simulink model "Simulation"  (R2021b)
settings: Solver=FixedStepAuto  StartTime=0.0  StopTime=30  FixedStep=Ts  RelTol=1e-3
InitFcn:
  | Tf = 200;
  | Ts = 0.01;
  | T = 0:Ts:Tf;
  | rolla = T';
  | omegaa=T';
  | omegax =T';
  | %%
  | 
  | load('A');
  | A = A(2001:2000+length(T),:);
  | rolla(:,2) = A(:,2)-0.0661;
  | omegaa(:,2) = A(:,1);
  | omegax(:,2) = A(:,3);
  | %%
  | l1 =10;
  | initial_vector_error = ones(1,l1)*0.001;
  | initial_vector_error(1) = 0.001;
undefined symbols (not defined in the file or in its folder): X, Y, Z
libraries: nesl_utility x23, sm_lib x15, simulink x3
(part 1 of 2)
settings Model: Creator=mirha  LastModifiedBy=Ali
settings SolverCC: AlgebraicLoopSolver=TrustRegion
settings DataIOCC: ReturnWorkspaceOutputs=off
settings DebuggingCC: SFMachineParentedDataDiag=warning  ArithmeticOperatorsInVariantConditions=warning
settings SFSimCC: SimUseLocalCustomCode=off  CustomCodeUndefinedFunction=UseInterfaceOnly
settings RTWCC: RTWUseLocalCustomCode=off

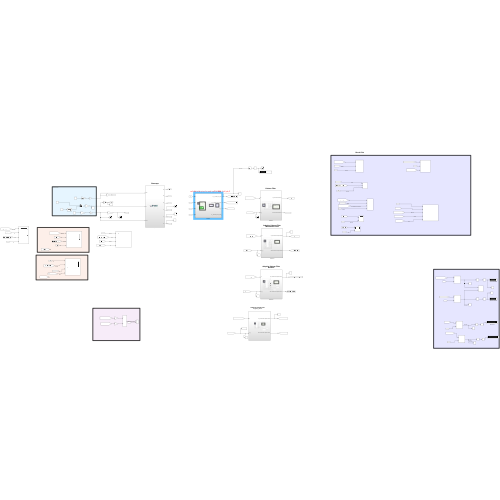
[thumbnail: Simulink's stored preview of the top-level diagram]
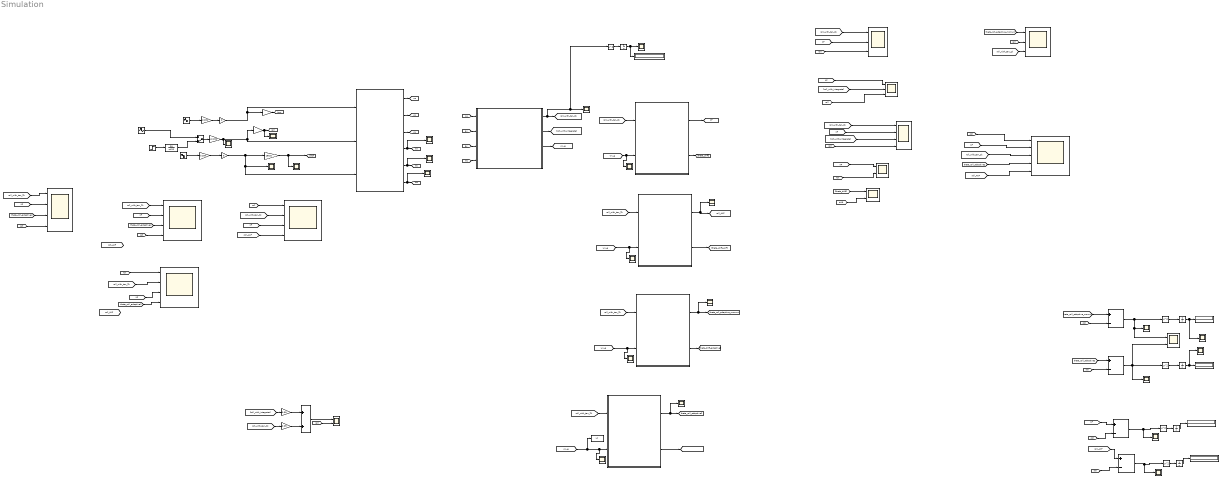
== system Simulation ==
  note: RMS error
  note: Result plot
  note: Kalman Filter
  note: اثر نویز که از IMA اندازگیری کردیم رو توی این بلوک اضافه شده
  note: plot
  note: Desired theta
  note: Result Plot
  note: Simscape
  note: Adaptive Kalman Filter
      | Momuni
  note: Adaptive Kalman Filter
      | Mohammad 1999
  note: Adaptive Kalman Filter
      | forgetting factor
  Display : Display
  Gain : Gain  Gain=0
  Gain1 : Gain  Gain=pi/180
  Gain11 : Gain  Gain=0
  Gain2 : Gain  Gain=180/pi
  Gain3 : Gain  Gain=180/pi
  Gain4 : Gain  Gain=0.95
  Gain5 : Gain  Gain=0.05
  Gain6 : Gain  Gain=pi/180
  Gain7 : Gain  Gain=pi/180
  Gain8 : Gain  Gain=180/pi
  Integrator{,1..4} (5 alike) : Integrator
  Kalma filter : Subsystem
  Kalma filter1 : Subsystem
  Kalma filter2 : Subsystem
  Kalma filter3 : Subsystem
  Manual Switch : ManualSwitch  CurrentSetting=0
  Math Function{,1..4} (5 alike) : Math  Operator=square  SignedPower=on  SaturateOnIntegerOverflow=on
  RMS error KF : Display
  RMS error KF1 : Display
  RMS error MOMUNI : Display
  RMS error1 FF AKF : Display
  Scope{,3,5,7,11,13..15,17..20,22..26,28..30,33..34} (22 alike) : Scope
  Scope{1,9,16,31..32} (5 alike) : Scope  NumInputPorts=4
  Scope10 : Scope  NumInputPorts=3
  Scope{2,4,12,21} (4 alike) : Scope  NumInputPorts=2
  Scope27 : Scope  NumInputPorts=5
  Scope6 : Scope  NumInputPorts=3
  Scope8 : Scope  NumInputPorts=3
  Simscape Model : Subsystem
  Sine Wave1 : Sin  Amplitude=20  SampleTime=0
  Sine Wave2 : Sin  Amplitude=50  Frequency=0.05  SampleTime=0
  Sine Wave3 : Sin  Amplitude=40  SampleTime=0
  Step : Step  Time=10  After=50  SampleTime=0
  Sum{,1..2,4} (4 alike) : Sum  Inputs=+-
  Sum3 : Sum
  To Workspace1 : ToWorkspace  VariableName=uk  SampleTime=-1
  Transfer Fcn : TransferFcn  Numerator=[20]  Denominator=[1 20]
  mosalasati : Subsystem
  tag scope: KF=global, Yaw=global, ax=global, ay=global, az=global, pitch=global, roll=global, roll_AKF=global, roll_with_tan_Zk=global, theta_roll_adaptive2=global, theta_roll_adaptive_momuni=global, wx=global, wx_g=global, wy=global, wz=global
  wires:
  Gain1/1 -> Gain/1
  Gain2/1 -> Scope/1, [roll]
  Gain/1 -> Simscape Model/1(YAW), Gain8/1
  Gain11/1 -> Scope26/1, Simscape Model/3(PItch), Gain3/1
  Sine Wave3/1 -> Gain7/1
  Gain6/1 -> Scope13/1, Simscape Model/2("roll "), Gain2/1
  Sine Wave2/1 -> Gain1/1
  Gain7/1 -> Gain11/1
  Simscape Model/2(Wx) -> [wx]
  Simscape Model/4(ax) -> Scope17/1, [ax]
  Simscape Model/5(ay) -> Scope24/1, [ay]
  Simscape Model/6(az) -> Scope25/1, [az]
  [roll] -> Scope2/2  "actual roll"
  Gain5/1 -> Sum3/2
  [roll_with_integrate] -> Gain4/1
  [roll_with_tan_Zk] -> Gain5/1
  Sum3/1 -> Scope2/1  "calculated with 95% and 5%"
  Gain4/1 -> Sum3/1
  Gain8/1 -> [Yaw]
  mosalasati/3(wx_g) -> [wx_g]
  [wx_g] -> Scope5/1, Kalma filter/2(wx_g)
  [roll_with_tan_Zk] -> Kalma filter/1(Zk)
  [roll_with_tan_Zk] -> Scope6/1  "Acc"
  [KF] -> Scope6/2  "kalman"
  [roll] -> Scope8/3  "actual roll"
  [KF] -> Scope8/1  "kalman"
  [roll] -> Scope6/3  "actual roll"
  [roll_with_integrate] -> Scope8/2  "roll calculatef with wx(integral)"
  Kalma filter/1(roll_calculated with Kalman) -> [KF]
  [KF] -> Scope4/1  "kalman"
  [roll] -> Scope4/2  "actual roll"
  [theta_drift] -> Scope12/1  "drift kalman"
  [drift] -> Scope12/2  "drift"
  Kalma filter/2(drift calculated with Kalman) -> [theta_drift]
  mosalasati/2(roll__calculated_with_integrat) -> [roll_with_integrate]
  [KF] -> Scope9/2  "kalman"
  [roll_with_tan_Zk] -> Scope9/1  "Acc"
  [roll_with_integrate] -> Scope9/3  "roll calculatef with wx(integral)"
  [roll] -> Scope9/4  "actual roll"
  [wx] -> mosalasati/1(wx)
  [ax] -> mosalasati/2(ax)
  [ay] -> mosalasati/3(ay)
  [az] -> mosalasati/4(az)
  Kalma filter1/2(drift calculated with adaptive Kalman) -> [theta_drift_adaptive]
  Kalma filter1/1(roll_calculated with adaptive Kalman) -> Scope11/1, [theta_roll_adaptive_momuni]
  [roll_with_tan_Zk] -> Kalma filter1/1(Zk)
  [wx_g] -> Kalma filter1/2(wx_g), Scope7/1
  [theta_roll_adaptive_momuni] -> Sum/1
  [roll] -> Sum/2
  [roll] -> Sum1/2
  [theta_roll_adaptive2] -> Sum1/1
  Sum/1 -> Scope21/1, Scope20/1, Math Function/1  "error momonu"
  Math Function/1 -> Integrator/1
  Integrator/1 -> Scope18/1, RMS error MOMUNI/1
  Integrator1/1 -> Scope22/1, RMS error1 FF AKF/1
  Math Function1/1 -> Integrator1/1
  Sum1/1 -> Scope21/2, Scope19/1, Math Function1/1  "error inv(R)"
  [KF] -> Sum2/1
  [roll] -> Sum2/2
  Sum2/1 -> Scope23/1, Math Function2/1  "error inv(R)"
  Math Function2/1 -> Integrator2/1
  Integrator2/1 -> RMS error KF/1
  Simscape Model/3(Wy) -> [wy]
  Simscape Model/1(Wz) -> [wz]
  [roll] -> Scope27/1  "actual roll"
  [KF] -> Scope27/2  "KF"
  [roll_with_tan_Zk] -> Scope27/3  "IMU raw"
  [theta_roll_adaptive2] -> Scope27/4  "FFAKF"
  [roll_with_tan_Zk] -> Kalma filter3/1(Zk)
  Kalma filter3/2(drift calculated with adaptive Kalman) -> [theta_drift_AKF]
  Kalma filter3/1(roll_calculated with adaptive Kalman) -> Scope28/1, [roll_AKF]
  [wx_g] -> Kalma filter3/2(wx_g), Scope29/1
  [theta_roll_adaptive_momuni] -> Scope10/1
  [roll] -> Scope10/2
  [roll_with_tan_Zk] -> Scope10/3
  [roll_AKF] -> Scope27/5  "AKF"
  Manual Switch/1 -> Gain6/1
  Transfer Fcn/1 -> Manual Switch/2
  Step/1 -> Transfer Fcn/1
  Sine Wave1/1 -> Manual Switch/1
  [roll] -> Scope16/1  "actual roll"
  [roll_with_tan_Zk] -> Scope16/2  "IMU"
  [KF] -> Scope16/3  "Kalman"
  Gain3/1 -> Scope30/1, [pitch]
  [roll_AKF] -> Scope16/4  "AKF"
  Kalma filter2/2(drift calculated with adaptive Kalman) -> [theta_drift_adaptive2]
  [roll_with_tan_Zk] -> Kalma filter2/1(Zk)
  Kalma filter2/1(roll_calculated with adaptive Kalman) -> [theta_roll_adaptive2], Scope14/1
  [wx_g] -> To Workspace1/1, Scope15/1, Kalma filter2/2(wx_g)
  [roll_with_tan_Zk] -> Scope1/1  "IMU data"
  [roll] -> Scope1/4  "Roll"
  [theta_roll_adaptive2] -> Scope1/3  "FFAKF"
  [KF] -> Scope1/2  "KF"
  [roll_with_tan_Zk] -> Scope32/1  "IMU data"
  [KF] -> Scope32/2  "KF"
  [theta_roll_adaptive2] -> Scope32/3  "FFAKF"
  [roll] -> Scope32/4  "Roll"
  [roll] -> Scope31/1  "Roll"
  [roll_with_tan_Zk] -> Scope31/2  "IMU data"
  [KF] -> Scope31/3  "KF"
  [theta_roll_adaptive2] -> Scope31/4  "FFAKF"
  mosalasati/1(roll__calculated_from_Acc) -> Math Function3/1, Scope3/1, [roll_with_tan_Zk]  "error inv(R)"
  Math Function3/1 -> Integrator3/1
  Integrator3/1 -> Display/1, Scope33/1
  [roll_AKF] -> Sum4/1
  [roll] -> Sum4/2
  Integrator4/1 -> RMS error KF1/1
  Math Function4/1 -> Integrator4/1
  Sum4/1 -> Math Function4/1, Scope34/1  "error inv(R)"

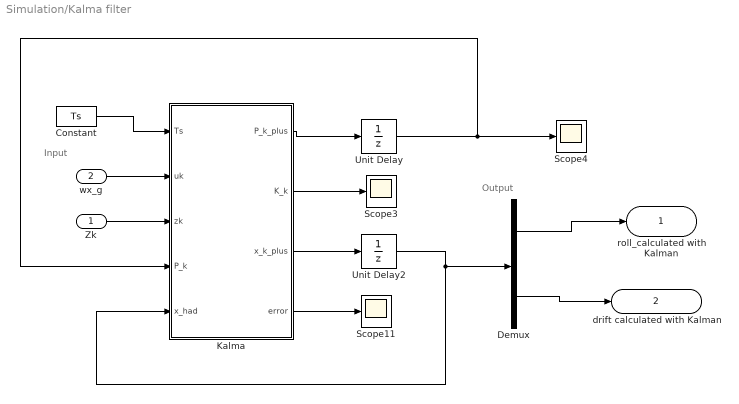
== system Simulation/Kalma filter ==
  note: Output
  note: Input
  Zk : Inport
  wx_g : Inport  Port=2
  Constant : Constant  Value=Ts
  Demux : Demux  Outputs=2
  Kalma : MATLAB Function  TreatAsAtomicUnit=on
  Scope11 : Scope
  Scope3 : Scope
  Scope4 : Scope
  Unit Delay : UnitDelay  InitialCondition=10*eye(2);  SampleTime=-1  HasFrameUpgradeWarning=on
  Unit Delay2 : UnitDelay  InitialCondition=[0;0.1]  SampleTime=-1  HasFrameUpgradeWarning=on
  roll_calculated with Kalman : Outport  VectorParamsAs1DForOutWhenUnconnected=off
  drift calculated with Kalman : Outport  Port=2  VectorParamsAs1DForOutWhenUnconnected=off
  wires:
  Kalma/4(error) -> Scope11/1
  Unit Delay/1 -> Kalma/4(P_k), Scope4/1
  Constant/1 -> Kalma/1(Ts)
  Kalma/1(P_k_plus) -> Unit Delay/1
  Kalma/3(x_k_plus) -> Unit Delay2/1
  Kalma/2(K_k) -> Scope3/1
  Unit Delay2/1 -> Kalma/5(x_had), Demux/1
  Zk/1 -> Kalma/3(zk)
  Demux/1 -> roll_calculated with Kalman/1
  Demux/2 -> drift calculated with Kalman/1
  wx_g/1 -> Kalma/2(uk)

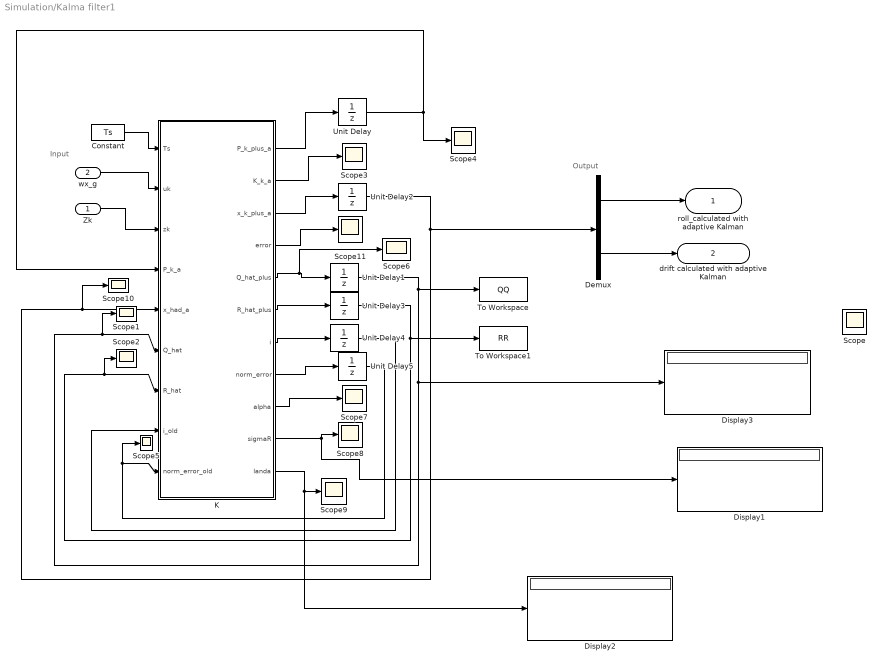
== system Simulation/Kalma filter1 ==
  note: Input
  note: Output
  Zk : Inport
  wx_g : Inport  Port=2
  Constant : Constant  Value=Ts
  Demux : Demux  Outputs=2
  Display1 : Display
  Display2 : Display
  Display3 : Display
  K : MATLAB Function  TreatAsAtomicUnit=on
  Scope{,1..11} (12 alike) : Scope
  To Workspace : ToWorkspace  VariableName=QQ  SampleTime=-1
  To Workspace1 : ToWorkspace  VariableName=RR  SampleTime=-1
  Unit Delay : UnitDelay  InitialCondition=10*eye(2);  SampleTime=-1  HasFrameUpgradeWarning=on
  Unit Delay1 : UnitDelay  InitialCondition=20*eye(2);  SampleTime=-1  HasFrameUpgradeWarning=on
  Unit Delay2 : UnitDelay  InitialCondition=[0;0.1]  SampleTime=-1  HasFrameUpgradeWarning=on
  Unit Delay3 : UnitDelay  InitialCondition=50  SampleTime=-1  HasFrameUpgradeWarning=on
  Unit Delay4 : UnitDelay  SampleTime=-1  HasFrameUpgradeWarning=on
  Unit Delay5 : UnitDelay  InitialCondition=0.001  SampleTime=-1  HasFrameUpgradeWarning=on
  roll_calculated with adaptive Kalman : Outport  VectorParamsAs1DForOutWhenUnconnected=off
  drift calculated with adaptive Kalman : Outport  Port=2  VectorParamsAs1DForOutWhenUnconnected=off
  wires:
  wx_g/1 -> K/2(uk)
  Demux/2 -> drift calculated with adaptive Kalman/1
  Demux/1 -> roll_calculated with adaptive Kalman/1
  Zk/1 -> K/3(zk)
  Unit Delay2/1 -> Scope10/1, K/5(x_had_a), Demux/1
  K/2(K_k_a) -> Scope3/1
  K/3(x_k_plus_a) -> Unit Delay2/1
  K/1(P_k_plus_a) -> Unit Delay/1
  Constant/1 -> K/1(Ts)
  Unit Delay/1 -> Scope4/1, K/4(P_k_a)
  K/4(error) -> Scope11/1
  K/5(Q_hat_plus) -> Scope6/1, Unit Delay1/1
  Unit Delay1/1 -> To Workspace/1, Display3/1, Scope1/1, K/6(Q_hat)
  K/6(R_hat_plus) -> Unit Delay3/1
  Unit Delay3/1 -> To Workspace1/1, Scope2/1, K/7(R_hat)
  K/7(i) -> Unit Delay4/1
  Unit Delay4/1 -> K/8(i_old)
  Unit Delay5/1 -> Scope5/1, K/9(norm_error_old)
  K/8(norm_error) -> Unit Delay5/1
  K/9(alpha) -> Scope7/1
  K/10(sigmaR) -> Scope8/1, Display1/1
  K/11(landa) -> Display2/1, Scope9/1

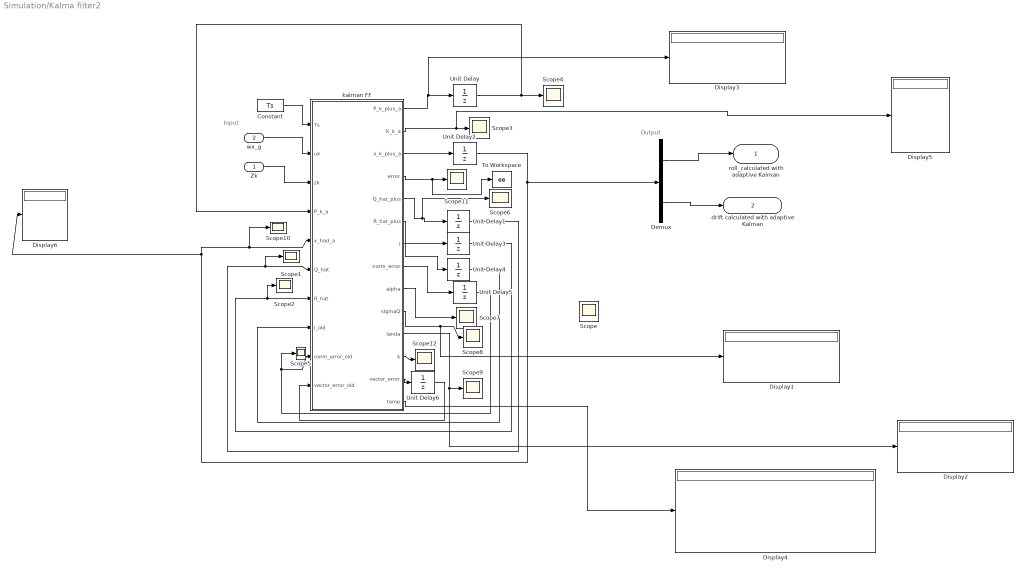
== system Simulation/Kalma filter2 ==
  note: Output
  note: Input
  Zk : Inport
  wx_g : Inport  Port=2
  Constant : Constant  Value=Ts
  Demux : Demux  Outputs=2
  Display{1..6} (6 alike) : Display
  Scope{,1..12} (13 alike) : Scope
  To Workspace : ToWorkspace  VariableName=ee  SampleTime=-1
  Unit Delay : UnitDelay  InitialCondition=0.01*eye(2);  SampleTime=-1  HasFrameUpgradeWarning=on
  Unit Delay1 : UnitDelay  InitialCondition=20*eye(2);  SampleTime=-1  HasFrameUpgradeWarning=on
  Unit Delay2 : UnitDelay  InitialCondition=[0;0.1]  SampleTime=-1  HasFrameUpgradeWarning=on
  Unit Delay3 : UnitDelay  InitialCondition=50  SampleTime=-1  HasFrameUpgradeWarning=on
  Unit Delay4 : UnitDelay  SampleTime=-1  HasFrameUpgradeWarning=on
  Unit Delay5 : UnitDelay  InitialCondition=0.001  SampleTime=-1  HasFrameUpgradeWarning=on
  Unit Delay6 : UnitDelay  InitialCondition=initial_vector_error  SampleTime=-1  HasFrameUpgradeWarning=on
  kalman FF : MATLAB Function  TreatAsAtomicUnit=on
  roll_calculated with adaptive Kalman : Outport  VectorParamsAs1DForOutWhenUnconnected=off
  drift calculated with adaptive Kalman : Outport  Port=2  VectorParamsAs1DForOutWhenUnconnected=off
  wires:
  kalman FF/11(landa) -> Display2/1, Scope9/1
  kalman FF/10(sigmaQ) -> Display1/1, Scope8/1
  kalman FF/9(alpha) -> Scope7/1
  kalman FF/8(norm_error) -> Unit Delay5/1
  Unit Delay5/1 -> kalman FF/9(norm_error_old), Scope5/1
  Unit Delay4/1 -> kalman FF/8(i_old)
  kalman FF/7(i) -> Unit Delay4/1
  Unit Delay3/1 -> kalman FF/7(R_hat), Scope2/1
  kalman FF/6(R_hat_plus) -> Unit Delay3/1
  Unit Delay1/1 -> kalman FF/6(Q_hat), Scope1/1
  kalman FF/5(Q_hat_plus) -> Unit Delay1/1, Scope6/1
  kalman FF/4(error) -> To Workspace/1, Scope11/1
  Unit Delay/1 -> kalman FF/4(P_k_a), Scope4/1
  Constant/1 -> kalman FF/1(Ts)
  kalman FF/1(P_k_plus_a) -> Display3/1, Unit Delay/1
  kalman FF/3(x_k_plus_a) -> Unit Delay2/1
  kalman FF/2(K_k_a) -> Display5/1, Scope3/1
  Unit Delay2/1 -> Demux/1, Display6/1, kalman FF/5(x_had_a), Scope10/1
  Zk/1 -> kalman FF/3(zk)
  Demux/1 -> roll_calculated with adaptive Kalman/1
  Demux/2 -> drift calculated with adaptive Kalman/1
  wx_g/1 -> kalman FF/2(uk)
  kalman FF/13(vector_error) -> Unit Delay6/1
  Unit Delay6/1 -> kalman FF/10(vector_error_old)
  kalman FF/12(k) -> Scope12/1
  kalman FF/14(temp) -> Display4/1

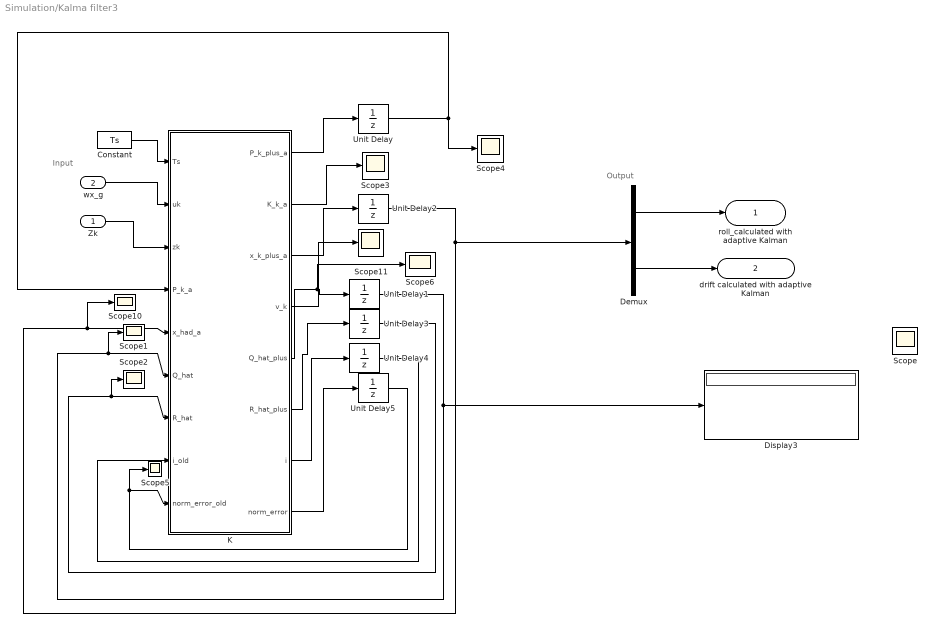
== system Simulation/Kalma filter3 ==
  note: Input
  note: Output
  Zk : Inport
  wx_g : Inport  Port=2
  Constant : Constant  Value=Ts
  Demux : Demux  Outputs=2
  Display3 : Display
  K : MATLAB Function  TreatAsAtomicUnit=on
  Scope{,1..6,10..11} (9 alike) : Scope
  Unit Delay : UnitDelay  InitialCondition=10*eye(2);  SampleTime=-1  HasFrameUpgradeWarning=on
  Unit Delay1 : UnitDelay  InitialCondition=20*eye(2);  SampleTime=-1  HasFrameUpgradeWarning=on
  Unit Delay2 : UnitDelay  InitialCondition=[0;0.1]  SampleTime=-1  HasFrameUpgradeWarning=on
  Unit Delay3 : UnitDelay  InitialCondition=50  SampleTime=-1  HasFrameUpgradeWarning=on
  Unit Delay4 : UnitDelay  SampleTime=-1  HasFrameUpgradeWarning=on
  Unit Delay5 : UnitDelay  InitialCondition=0.001  SampleTime=-1  HasFrameUpgradeWarning=on
  roll_calculated with adaptive Kalman : Outport  VectorParamsAs1DForOutWhenUnconnected=off
  drift calculated with adaptive Kalman : Outport  Port=2  VectorParamsAs1DForOutWhenUnconnected=off
  wires:
  wx_g/1 -> K/2(uk)
  Demux/2 -> drift calculated with adaptive Kalman/1
  Demux/1 -> roll_calculated with adaptive Kalman/1
  Zk/1 -> K/3(zk)
  Unit Delay2/1 -> Scope10/1, K/5(x_had_a), Demux/1
  K/2(K_k_a) -> Scope3/1
  K/3(x_k_plus_a) -> Unit Delay2/1
  K/1(P_k_plus_a) -> Unit Delay/1
  Constant/1 -> K/1(Ts)
  Unit Delay/1 -> Scope4/1, K/4(P_k_a)
  K/4(v_k) -> Scope11/1
  K/5(Q_hat_plus) -> Scope6/1, Unit Delay1/1
  Unit Delay1/1 -> Display3/1, Scope1/1, K/6(Q_hat)
  K/6(R_hat_plus) -> Unit Delay3/1
  Unit Delay3/1 -> Scope2/1, K/7(R_hat)
  K/7(i) -> Unit Delay4/1
  Unit Delay4/1 -> K/8(i_old)
  Unit Delay5/1 -> Scope5/1, K/9(norm_error_old)
  K/8(norm_error) -> Unit Delay5/1

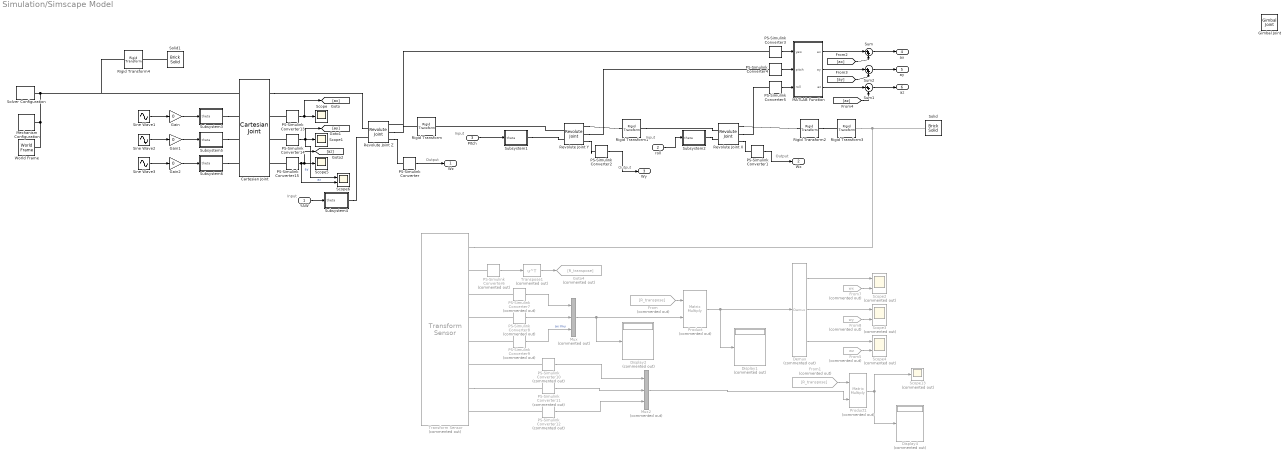
== system Simulation/Simscape Model ==
  note: Output
  note: Output
  note: Output
  note: Input
  note: Input
  note: Input
  YAW : Inport
  "roll " : Inport  Port=2
  PItch : Inport  Port=3
  Cartesian Joint : sm_lib/Joints/Cartesian Joint  JointMode=Normal  SenseConstraintForce=off  SenseConstraintForceX=off  SenseConstraintForceY=off  SenseConstraintForceZ=off  SenseConstraintTorque=off  SenseConstraintTorqueX=off  SenseConstraintTorqueY=off  SenseConstraintTorqueZ=off  SenseTotalForce=off  SenseTotalForceX=off  SenseTotalForceY=off  SenseTotalForceZ=off  SenseTotalTorque=off  SenseTotalTorqueX=off  SenseTotalTorqueY=off  SenseTotalTorqueZ=off  CompositeWrenchDir=FollowerOnBase  CompositeWrenchFrame=BaseFrame  PxEquilibriumPosition=0  PxEquilibriumPositionUnits=m  PxSpringStiffness=0  PxSpringStiffnessUnits=N/m  PxDampingCoefficient=0  PxDampingCoefficientUnits=N/(m/s)  PxTorqueActuationMode=ComputedTorque  PxMotionActuationMode=InputMotion  PxSensePosition=off  PxSenseVelocity=off  PxSenseAcceleration=on  PxSenseTorqueForce=off  PxSenseLowerLimitTorqueForce=off  PxSenseUpperLimitTorqueForce=off  PxLowerLimitSpecify=off  PxLowerLimitBound=-1  PxLowerLimitBoundUnits=m  PxLowerLimitStiffness=1e6  PxLowerLimitStiffnessUnits=N/m  PxLowerLimitDamping=1e3  PxLowerLimitDampingUnits=N/(m/s)  PxLowerLimitTransitionRegionWidth=1e-4  PxLowerLimitTransitionRegionWidthUnits=m  PxUpperLimitSpecify=off  PxUpperLimitBound=1  PxUpperLimitBoundUnits=m  PxUpperLimitStiffness=1e6  PxUpperLimitStiffnessUnits=N/m  PxUpperLimitDamping=1e3  PxUpperLimitDampingUnits=N/(m/s)  PxUpperLimitTransitionRegionWidth=1e-4  PxUpperLimitTransitionRegionWidthUnits=m  PxPositionTargetSpecify=off  PxPositionTargetPriority=High  PxPositionTargetValue=0  PxPositionTargetValueUnits=m  PxVelocityTargetSpecify=off  PxVelocityTargetPriority=High  PxVelocityTargetValue=0  PxVelocityTargetValueUnits=m/s  PyEquilibriumPosition=0  PyEquilibriumPositionUnits=m  PySpringStiffness=0  PySpringStiffnessUnits=N/m  PyDampingCoefficient=0  PyDampingCoefficientUnits=N/(m/s)  PyTorqueActuationMode=ComputedTorque  PyMotionActuationMode=InputMotion  PySensePosition=off  PySenseVelocity=off  PySenseAcceleration=on  PySenseTorqueForce=off  PySenseLowerLimitTorqueForce=off  PySenseUpperLimitTorqueForce=off  PyLowerLimitSpecify=off  PyLowerLimitBound=-1  PyLowerLimitBoundUnits=m  PyLowerLimitStiffness=1e6  PyLowerLimitStiffnessUnits=N/m  PyLowerLimitDamping=1e3  PyLowerLimitDampingUnits=N/(m/s)  PyLowerLimitTransitionRegionWidth=1e-4  PyLowerLimitTransitionRegionWidthUnits=m  PyUpperLimitSpecify=off  PyUpperLimitBound=1  PyUpperLimitBoundUnits=m  PyUpperLimitStiffness=1e6  PyUpperLimitStiffnessUnits=N/m  PyUpperLimitDamping=1e3  PyUpperLimitDampingUnits=N/(m/s)  PyUpperLimitTransitionRegionWidth=1e-4  PyUpperLimitTransitionRegionWidthUnits=m  PyPositionTargetSpecify=off  PyPositionTargetPriority=High  PyPositionTargetValue=0  PyPositionTargetValueUnits=m  PyVelocityTargetSpecify=off  PyVelocityTargetPriority=High  PyVelocityTargetValue=0  PyVelocityTargetValueUnits=m/s  PzEquilibriumPosition=0  PzEquilibriumPositionUnits=m  PzSpringStiffness=0  PzSpringStiffnessUnits=N/m  PzDampingCoefficient=0  PzDampingCoefficientUnits=N/(m/s)  PzTorqueActuationMode=ComputedTorque  PzMotionActuationMode=InputMotion  PzSensePosition=off  PzSenseVelocity=off  PzSenseAcceleration=on  PzSenseTorqueForce=off  PzSenseLowerLimitTorqueForce=off  PzSenseUpperLimitTorqueForce=off  PzLowerLimitSpecify=off  PzLowerLimitBound=-1  PzLowerLimitBoundUnits=m  PzLowerLimitStiffness=1e6  PzLowerLimitStiffnessUnits=N/m  PzLowerLimitDamping=1e3  PzLowerLimitDampingUnits=N/(m/s)  PzLowerLimitTransitionRegionWidth=1e-4  PzLowerLimitTransitionRegionWidthUnits=m  PzUpperLimitSpecify=off  PzUpperLimitBound=1  PzUpperLimitBoundUnits=m  PzUpperLimitStiffness=1e6  PzUpperLimitStiffnessUnits=N/m  PzUpperLimitDamping=1e3  PzUpperLimitDampingUnits=N/(m/s)  PzUpperLimitTransitionRegionWidth=1e-4  PzUpperLimitTransitionRegionWidthUnits=m  PzPositionTargetSpecify=off  PzPositionTargetPriority=High  PzPositionTargetValue=0  PzPositionTargetValueUnits=m  PzVelocityTargetSpecify=off  PzVelocityTargetPriority=High  PzVelocityTargetValue=0  PzVelocityTargetValueUnits=m/s
  Demux : Demux  Commented=on  Outputs=3
  Display1 : Display  Commented=on
  Display2 : Display  Commented=on
  Display4 : Display  Commented=on
  From : From  Commented=on  GotoTag=R_transpose
  From1 : From  Commented=on  GotoTag=R_transpose
  From5 : From  Commented=on  GotoTag=wz
  From7 : From  Commented=on  GotoTag=wx  TagVisibility=global
  From8 : From  Commented=on  GotoTag=wy
  Gain : Gain  Gain=0
  Gain1 : Gain  Gain=0
  Gain2 : Gain  Gain=0
  Gimbal Joint : sm_lib/Joints/Gimbal Joint  JointMode=Normal  SenseConstraintForce=off  SenseConstraintForceX=off  SenseConstraintForceY=off  SenseConstraintForceZ=off  SenseConstraintTorque=off  SenseConstraintTorqueX=off  SenseConstraintTorqueY=off  SenseConstraintTorqueZ=off  SenseTotalForce=off  SenseTotalForceX=off  SenseTotalForceY=off  SenseTotalForceZ=off  SenseTotalTorque=off  SenseTotalTorqueX=off  SenseTotalTorqueY=off  SenseTotalTorqueZ=off  CompositeWrenchDir=FollowerOnBase  CompositeWrenchFrame=BaseFrame  RxEquilibriumPosition=0  RxEquilibriumPositionUnits=deg  RxSpringStiffness=0  RxSpringStiffnessUnits=N*m/deg  RxDampingCoefficient=0  RxDampingCoefficientUnits=N*m/(deg/s)  RxTorqueActuationMode=NoTorque  RxMotionActuationMode=ComputedMotion  RxSensePosition=off  RxSenseVelocity=off  RxSenseAcceleration=off  RxSenseTorqueForce=off  RxSenseLowerLimitTorqueForce=off  RxSenseUpperLimitTorqueForce=off  RxLowerLimitSpecify=off  RxLowerLimitBound=-90  RxLowerLimitBoundUnits=deg  RxLowerLimitStiffness=1e4  RxLowerLimitStiffnessUnits=N*m/deg  RxLowerLimitDamping=10  RxLowerLimitDampingUnits=N*m/(deg/s)  RxLowerLimitTransitionRegionWidth=0.1  RxLowerLimitTransitionRegionWidthUnits=deg  RxUpperLimitSpecify=off  RxUpperLimitBound=90  RxUpperLimitBoundUnits=deg  RxUpperLimitStiffness=1e4  RxUpperLimitStiffnessUnits=N*m/deg  RxUpperLimitDamping=10  RxUpperLimitDampingUnits=N*m/(deg/s)  RxUpperLimitTransitionRegionWidth=0.1  RxUpperLimitTransitionRegionWidthUnits=deg  RxPositionTargetSpecify=off  RxPositionTargetPriority=High  RxPositionTargetValue=0  RxPositionTargetValueUnits=deg  RxVelocityTargetSpecify=off  RxVelocityTargetPriority=High  RxVelocityTargetValue=0  RxVelocityTargetValueUnits=deg/s  RyEquilibriumPosition=0  RyEquilibriumPositionUnits=deg  RySpringStiffness=0  RySpringStiffnessUnits=N*m/deg  RyDampingCoefficient=0  RyDampingCoefficientUnits=N*m/(deg/s)  RyTorqueActuationMode=NoTorque  RyMotionActuationMode=ComputedMotion  RySensePosition=off  RySenseVelocity=off  RySenseAcceleration=off  RySenseTorqueForce=off  RySenseLowerLimitTorqueForce=off  RySenseUpperLimitTorqueForce=off  RyLowerLimitSpecify=off  RyLowerLimitBound=-90  RyLowerLimitBoundUnits=deg  RyLowerLimitStiffness=1e4  RyLowerLimitStiffnessUnits=N*m/deg  RyLowerLimitDamping=10  RyLowerLimitDampingUnits=N*m/(deg/s)  RyLowerLimitTransitionRegionWidth=0.1  RyLowerLimitTransitionRegionWidthUnits=deg  RyUpperLimitSpecify=off  RyUpperLimitBound=90  RyUpperLimitBoundUnits=deg  RyUpperLimitStiffness=1e4  RyUpperLimitStiffnessUnits=N*m/deg  RyUpperLimitDamping=10  RyUpperLimitDampingUnits=N*m/(deg/s)  RyUpperLimitTransitionRegionWidth=0.1  RyUpperLimitTransitionRegionWidthUnits=deg  RyPositionTargetSpecify=off  RyPositionTargetPriority=High  RyPositionTargetValue=0  RyPositionTargetValueUnits=deg  RyVelocityTargetSpecify=off  RyVelocityTargetPriority=High  RyVelocityTargetValue=0  RyVelocityTargetValueUnits=deg/s  RzEquilibriumPosition=0  RzEquilibriumPositionUnits=deg  RzSpringStiffness=0  RzSpringStiffnessUnits=N*m/deg  RzDampingCoefficient=0  RzDampingCoefficientUnits=N*m/(deg/s)  RzTorqueActuationMode=NoTorque  RzMotionActuationMode=ComputedMotion  RzSensePosition=off  RzSenseVelocity=off  RzSenseAcceleration=off  RzSenseTorqueForce=off  RzSenseLowerLimitTorqueForce=off  RzSenseUpperLimitTorqueForce=off  RzLowerLimitSpecify=off  RzLowerLimitBound=-90  RzLowerLimitBoundUnits=deg  RzLowerLimitStiffness=1e4  RzLowerLimitStiffnessUnits=N*m/deg  RzLowerLimitDamping=10  RzLowerLimitDampingUnits=N*m/(deg/s)  RzLowerLimitTransitionRegionWidth=0.1  RzLowerLimitTransitionRegionWidthUnits=deg  RzUpperLimitSpecify=off  RzUpperLimitBound=90  RzUpperLimitBoundUnits=deg  RzUpperLimitStiffness=1e4  RzUpperLimitStiffnessUnits=N*m/deg  RzUpperLimitDamping=10  RzUpperLimitDampingUnits=N*m/(deg/s)  RzUpperLimitTransitionRegionWidth=0.1  RzUpperLimitTransitionRegionWidthUnits=deg  RzPositionTargetSpecify=off  RzPositionTargetPriority=High  RzPositionTargetValue=0  RzPositionTargetValueUnits=deg  RzVelocityTargetSpecify=off  RzVelocityTargetPriority=High  RzVelocityTargetValue=0  RzVelocityTargetValueUnits=deg/s
  Goto4 : Goto  Commented=on  GotoTag=R_transpose
  MATLAB Function : MATLAB Function  TreatAsAtomicUnit=on
  Mechanism Configuration : sm_lib/Utilities/Mechanism Configuration  UniformGravity=Constant  GravityVector=[0 0 -0]  GravityUnits=m/s^2  LinearizationDelta=0.001  JointModeTransitionNonlinearIterations=2
  Mux : Mux  Commented=on  Inputs=3
  Mux2 : Mux  Commented=on  Inputs=3
  PS-Simulink Converter{,1..5,13..15} (9 alike) : nesl_utility/PS-Simulink Converter  PhysicalDomain=network_engine_domain  SubClassName=ps_output  LeftPortType=input  RightPortType=output  PseudoPeriodic=off  Frequencies=[]  Unit=1  AffineConversion=off
      settings: SourceProductBaseCode=PW,SS
  PS-Simulink Converter{6..12} (7 alike) : nesl_utility/PS-Simulink Converter  Commented=on  PhysicalDomain=network_engine_domain  SubClassName=ps_output  LeftPortType=input  RightPortType=output  PseudoPeriodic=off  Frequencies=[]  Unit=1  AffineConversion=off
      settings: SourceProductBaseCode=PW,SS
  Product : Product  Commented=on  Multiplication=Matrix(*)
  Product1 : Product  Commented=on  Multiplication=Matrix(*)
  Revolute Joint X : sm_lib/Joints/Revolute Joint  JointMode=Normal  SenseConstraintForce=off  SenseConstraintForceX=off  SenseConstraintForceY=off  SenseConstraintForceZ=off  SenseConstraintTorque=off  SenseConstraintTorqueX=off  SenseConstraintTorqueY=off  SenseConstraintTorqueZ=off  SenseTotalForce=off  SenseTotalForceX=off  SenseTotalForceY=off  SenseTotalForceZ=off  SenseTotalTorque=off  SenseTotalTorqueX=off  SenseTotalTorqueY=off  SenseTotalTorqueZ=off  CompositeWrenchDir=FollowerOnBase  CompositeWrenchFrame=BaseFrame  EquilibriumPosition=0  EquilibriumPositionUnits=deg  SpringStiffness=0  SpringStiffnessUnits=N*m/deg  DampingCoefficient=0  DampingCoefficientUnits=N*m/(deg/s)  TorqueActuationMode=ComputedTorque  MotionActuationMode=InputMotion  SensePosition=on  SenseVelocity=on  SenseAcceleration=off  SenseTorqueForce=off  SenseLowerLimitTorqueForce=off  SenseUpperLimitTorqueForce=off  LowerLimitSpecify=off  LowerLimitBound=-90  LowerLimitBoundUnits=deg  LowerLimitStiffness=1e4  LowerLimitStiffnessUnits=N*m/deg  LowerLimitDamping=10  LowerLimitDampingUnits=N*m/(deg/s)  LowerLimitTransitionRegionWidth=0.1  LowerLimitTransitionRegionWidthUnits=deg  UpperLimitSpecify=off  UpperLimitBound=90  UpperLimitBoundUnits=deg  UpperLimitStiffness=1e4  UpperLimitStiffnessUnits=N*m/deg  UpperLimitDamping=10  UpperLimitDampingUnits=N*m/(deg/s)  UpperLimitTransitionRegionWidth=0.1  UpperLimitTransitionRegionWidthUnits=deg  PositionTargetSpecify=off  PositionTargetPriority=High  PositionTargetValue=0  PositionTargetValueUnits=deg  VelocityTargetSpecify=off  VelocityTargetPriority=High  VelocityTargetValue=0  VelocityTargetValueUnits=deg/s
  Revolute Joint Y : sm_lib/Joints/Revolute Joint  JointMode=Normal  SenseConstraintForce=off  SenseConstraintForceX=off  SenseConstraintForceY=off  SenseConstraintForceZ=off  SenseConstraintTorque=off  SenseConstraintTorqueX=off  SenseConstraintTorqueY=off  SenseConstraintTorqueZ=off  SenseTotalForce=off  SenseTotalForceX=off  SenseTotalForceY=off  SenseTotalForceZ=off  SenseTotalTorque=off  SenseTotalTorqueX=off  SenseTotalTorqueY=off  SenseTotalTorqueZ=off  CompositeWrenchDir=FollowerOnBase  CompositeWrenchFrame=BaseFrame  EquilibriumPosition=0  EquilibriumPositionUnits=deg  SpringStiffness=0  SpringStiffnessUnits=N*m/deg  DampingCoefficient=0  DampingCoefficientUnits=N*m/(deg/s)  TorqueActuationMode=ComputedTorque  MotionActuationMode=InputMotion  SensePosition=on  SenseVelocity=on  SenseAcceleration=off  SenseTorqueForce=off  SenseLowerLimitTorqueForce=off  SenseUpperLimitTorqueForce=off  LowerLimitSpecify=off  LowerLimitBound=-90  LowerLimitBoundUnits=deg  LowerLimitStiffness=1e4  LowerLimitStiffnessUnits=N*m/deg  LowerLimitDamping=10  LowerLimitDampingUnits=N*m/(deg/s)  LowerLimitTransitionRegionWidth=0.1  LowerLimitTransitionRegionWidthUnits=deg  UpperLimitSpecify=off  UpperLimitBound=90  UpperLimitBoundUnits=deg  UpperLimitStiffness=1e4  UpperLimitStiffnessUnits=N*m/deg  UpperLimitDamping=10  UpperLimitDampingUnits=N*m/(deg/s)  UpperLimitTransitionRegionWidth=0.1  UpperLimitTransitionRegionWidthUnits=deg  PositionTargetSpecify=off  PositionTargetPriority=High  PositionTargetValue=0  PositionTargetValueUnits=deg  VelocityTargetSpecify=off  VelocityTargetPriority=High  VelocityTargetValue=0  VelocityTargetValueUnits=deg/s
  Revolute Joint Z : sm_lib/Joints/Revolute Joint  JointMode=Normal  SenseConstraintForce=off  SenseConstraintForceX=off  SenseConstraintForceY=off  SenseConstraintForceZ=off  SenseConstraintTorque=off  SenseConstraintTorqueX=off  SenseConstraintTorqueY=off  SenseConstraintTorqueZ=off  SenseTotalForce=off  SenseTotalForceX=off  SenseTotalForceY=off  SenseTotalForceZ=off  SenseTotalTorque=off  SenseTotalTorqueX=off  SenseTotalTorqueY=off  SenseTotalTorqueZ=off  CompositeWrenchDir=FollowerOnBase  CompositeWrenchFrame=BaseFrame  EquilibriumPosition=0  EquilibriumPositionUnits=deg  SpringStiffness=0  SpringStiffnessUnits=N*m/deg  DampingCoefficient=0  DampingCoefficientUnits=N*m/(deg/s)  TorqueActuationMode=ComputedTorque  MotionActuationMode=InputMotion  SensePosition=on  SenseVelocity=on  SenseAcceleration=off  SenseTorqueForce=off  SenseLowerLimitTorqueForce=off  SenseUpperLimitTorqueForce=off  LowerLimitSpecify=off  LowerLimitBound=-90  LowerLimitBoundUnits=deg  LowerLimitStiffness=1e4  LowerLimitStiffnessUnits=N*m/deg  LowerLimitDamping=10  LowerLimitDampingUnits=N*m/(deg/s)  LowerLimitTransitionRegionWidth=0.1  LowerLimitTransitionRegionWidthUnits=deg  UpperLimitSpecify=off  UpperLimitBound=90  UpperLimitBoundUnits=deg  UpperLimitStiffness=1e4  UpperLimitStiffnessUnits=N*m/deg  UpperLimitDamping=10  UpperLimitDampingUnits=N*m/(deg/s)  UpperLimitTransitionRegionWidth=0.1  UpperLimitTransitionRegionWidthUnits=deg  PositionTargetSpecify=off  PositionTargetPriority=High  PositionTargetValue=0  PositionTargetValueUnits=deg  VelocityTargetSpecify=off  VelocityTargetPriority=High  VelocityTargetValue=0  VelocityTargetValueUnits=deg/s
  Rigid Transform : sm_lib/Frames and Transforms/Rigid Transform  TranslationMethod=None  TranslationStandardOffset=0  TranslationLengthUnit=m  TranslationStandardAxis=+Z  TranslationCartesianOffset=[0 0 0]  TranslationROffset=0  TranslationROffsetUnits=m  TranslationZOffset=0  TranslationZOffsetUnits=m  TranslationThetaOffset=0  TranslationThetaOffsetUnits=deg  RotationMethod=StandardAxis  RotationAngleUnits=deg  RotationStandardAxis=+X  RotationAngle=-90  RotationArbitraryAxis=[0 0 1]  FollAlignAxisA=+X  BaseAlignAxisA=+Y  FollAlignAxisB=+Y  BaseAlignAxisB=+Z  RotationSequenceAxes=FollowerAxes  RotationSequence=XYX  RotationSequenceAngles=[0 0 0]  RotationSequenceAnglesUnits=deg  RotationMatrix=[1 0 0; 0 1 0; 0 0 1]
  Rigid Transform1 : sm_lib/Frames and Transforms/Rigid Transform  TranslationMethod=None  TranslationStandardOffset=0  TranslationLengthUnit=m  TranslationStandardAxis=+Z  TranslationCartesianOffset=[0 0 0]  TranslationROffset=0  TranslationROffsetUnits=m  TranslationZOffset=0  TranslationZOffsetUnits=m  TranslationThetaOffset=0  TranslationThetaOffsetUnits=deg  RotationMethod=StandardAxis  RotationAngleUnits=deg  RotationStandardAxis=+Y  RotationAngle=90  RotationArbitraryAxis=[0 0 1]  FollAlignAxisA=+X  BaseAlignAxisA=+Y  FollAlignAxisB=+Y  BaseAlignAxisB=+Z  RotationSequenceAxes=FollowerAxes  RotationSequence=XYX  RotationSequenceAngles=[0 0 0]  RotationSequenceAnglesUnits=deg  RotationMatrix=[1 0 0; 0 1 0; 0 0 1]
  Rigid Transform2 : sm_lib/Frames and Transforms/Rigid Transform  TranslationMethod=None  TranslationStandardOffset=0  TranslationLengthUnit=m  TranslationStandardAxis=+Z  TranslationCartesianOffset=[0 0 0]  TranslationROffset=0  TranslationROffsetUnits=m  TranslationZOffset=0  TranslationZOffsetUnits=m  TranslationThetaOffset=0  TranslationThetaOffsetUnits=deg  RotationMethod=StandardAxis  RotationAngleUnits=deg  RotationStandardAxis=+X  RotationAngle=90  RotationArbitraryAxis=[0 0 1]  FollAlignAxisA=+X  BaseAlignAxisA=+Y  FollAlignAxisB=+Y  BaseAlignAxisB=+Z  RotationSequenceAxes=FollowerAxes  RotationSequence=XYX  RotationSequenceAngles=[0 0 0]  RotationSequenceAnglesUnits=deg  RotationMatrix=[1 0 0; 0 1 0; 0 0 1]
  Rigid Transform3 : sm_lib/Frames and Transforms/Rigid Transform  TranslationMethod=None  TranslationStandardOffset=0  TranslationLengthUnit=m  TranslationStandardAxis=+Z  TranslationCartesianOffset=[0 0 0]  TranslationROffset=0  TranslationROffsetUnits=m  TranslationZOffset=0  TranslationZOffsetUnits=m  TranslationThetaOffset=0  TranslationThetaOffsetUnits=deg  RotationMethod=StandardAxis  RotationAngleUnits=deg  RotationStandardAxis=+Z  RotationAngle=90  RotationArbitraryAxis=[0 0 1]  FollAlignAxisA=+X  BaseAlignAxisA=+Y  FollAlignAxisB=+Y  BaseAlignAxisB=+Z  RotationSequenceAxes=FollowerAxes  RotationSequence=XYX  RotationSequenceAngles=[0 0 0]  RotationSequenceAnglesUnits=deg  RotationMatrix=[1 0 0; 0 1 0; 0 0 1]
  Rigid Transform4 : sm_lib/Frames and Transforms/Rigid Transform  TranslationMethod=Cartesian  TranslationStandardOffset=0  TranslationLengthUnit=m  TranslationStandardAxis=+Z  TranslationCartesianOffset=[0 0 -0.005]  TranslationROffset=0  TranslationROffsetUnits=m  TranslationZOffset=0  TranslationZOffsetUnits=m  TranslationThetaOffset=0  TranslationThetaOffsetUnits=deg  RotationMethod=None  RotationAngleUnits=deg  RotationStandardAxis=+Y  RotationAngle=90  RotationArbitraryAxis=[0 0 1]  FollAlignAxisA=+X  BaseAlignAxisA=+Y  FollAlignAxisB=+Y  BaseAlignAxisB=+Z  RotationSequenceAxes=FollowerAxes  RotationSequence=XYX  RotationSequenceAngles=[0 0 0]  RotationSequenceAnglesUnits=deg  RotationMatrix=[1 0 0; 0 1 0; 0 0 1]
  Scope : Scope
  Scope1 : Scope
  Scope13 : Scope  Commented=on
  Scope2 : Scope  Commented=on  NumInputPorts=2
  Scope3 : Scope  Commented=on  NumInputPorts=2
  Scope4 : Scope  Commented=on  NumInputPorts=2
  Scope5 : Scope
  Scope6 : Scope  NumInputPorts=2
  Sine Wave1 : Sin  Amplitude=0.2  Frequency=3  SampleTime=0
  Sine Wave2 : Sin  Amplitude=0.02  SampleTime=0
  Sine Wave3 : Sin  Amplitude=0.02  Phase=90  SampleTime=0
  Solid : sm_lib/Body Elements/Brick Solid  GraphicAmbientColor=[0.15 0.15 0.15 1.0]  BasedOnType=Density  BrickDimensions=[1 1 1]  BrickDimensionUnits=cm  CenterOfMass=[0 0 0]  CenterOfMassUnits=m  GraphicDiffuseColor=[1.0 0.0 1.0]  Density=1000  DensityUnits=kg/m^3  DoExposeReferenceFrame=on  GraphicEmissiveColor=[0.0 0.0 0.0 1.0]  ExportEntireGeometry=off  SerializedFrames=<Frames/>  MarkerShape=Sphere  MarkerSize=10  GraphicType=FromGeometry  InertiaType=Custom  Mass=1  MassUnits=kg  MomentsOfInertia=[1 1 1]  MomentsOfInertiaUnits=kg*m^2  GraphicOpacity=1.0  ProductsOfInertia=[0 0 0]  ProductsOfInertiaUnits=kg*m^2  GraphicShininess=75  GraphicSpecularColor=[0.5 0.5 0.5 1.0]  GraphicVisPropType=SimpleVisualProperties
  Solid1 : sm_lib/Body Elements/Brick Solid  GraphicAmbientColor=[0.15 0.15 0.15 1.0]  BasedOnType=Density  BrickDimensions=[0.3 0.3 0.001]  BrickDimensionUnits=m  CenterOfMass=[0 0 0]  CenterOfMassUnits=m  GraphicDiffuseColor=[0.4 0.4 0.4]  Density=1000  DensityUnits=kg/m^3  DoExposeReferenceFrame=on  GraphicEmissiveColor=[0.0 0.0 0.0 1.0]  ExportEntireGeometry=off  SerializedFrames=<Frames/>  MarkerShape=Sphere  MarkerSize=10  GraphicType=FromGeometry  InertiaType=Custom  Mass=1  MassUnits=kg  MomentsOfInertia=[1 1 1]  MomentsOfInertiaUnits=kg*m^2  GraphicOpacity=1.0  ProductsOfInertia=[0 0 0]  ProductsOfInertiaUnits=kg*m^2  GraphicShininess=75  GraphicSpecularColor=[0.5 0.5 0.5 1.0]  GraphicVisPropType=SimpleVisualProperties
  Solver Configuration : nesl_utility/Solver Configuration  PhysicalDomain=network_engine_domain  SubClassName=solver  LeftPortType=input  RightPortType=generic  Tones=[]  Harmonics=[]  SimulateNoise=off  Profile=off  UseLocalSampling=off  EnableSwitchedLinearOptims=on  FrequencyDomain=off  UseCCode=off  RelTol=0.001  AbsTol=1e-06  MinStep=1e-09  ToWorkspace=off  RevertToSquareIcSolve=off  NumHomotopyIterations=100  PhasorMode=off  PhasorModeNumHarmonics=1  DoDC=off  ResidualTolerance=1e-09  UseLocalSolver=off  LocalSolverChoice=NE_BACKWARD_EULER_ADVANCER  LocalSolverSampleTime=0.001  DoFixedCost=off  MaxNonlinIter=3  MaxModeIter=2  ComputeImpulses=off  ImpulseIterations=2  LinearAlgebra=Sparse  EquationFormulation=NE_TIME_EF  DelaysMemoryBudget=1024  AutomaticFiltering=on  FilteringTimeConstant=0.001  PartitionStorageMethod=AS_NEEDED  PartitionMemoryBudget=1024  PartitionMethod=FAST
      settings: SourceProductBaseCode=PW,SS
  Subsystem1 : Subsystem
  Subsystem2 : Subsystem
  Subsystem3 : Subsystem
  Subsystem4 : Subsystem
  Subsystem5 : Subsystem
  Subsystem6 : Subsystem
  Sum : Sum  Inputs=|++
  Sum1 : Sum  Inputs=|++
  Sum2 : Sum  Inputs=|++
  Transform Sensor : sm_lib/Frames and Transforms/Transform Sensor  Commented=on  MeasurementFrame=World  SenseAngle=off  SenseAxis=off  SenseAngle1=off  SenseAngle2=off  SenseAngle3=off  SenseQ=off  SenseR=on  SenseOmegaX=on  SenseOmegaY=on  SenseOmegaZ=on  SenseOmega1=off  SenseOmega2=off  SenseOmega3=off  SenseQDot=off  SenseRDot=off  SenseAlphaX=off  SenseAlphaY=off  SenseAlphaZ=off  SenseAlpha1=off  SenseAlpha2=off  SenseAlpha3=off  SenseQDDot=off  SenseRDDot=off  SenseX=off  SenseY=off  SenseZ=off  SenseRad=off  SenseAzim=off  SenseDist=off  SenseInc=off  SenseXDot=off  SenseYDot=off  SenseZDot=off  SenseRadDot=off  SenseAzimDot=off  SenseDistDot=off  SenseIncDot=off  SenseXDDot=on  SenseYDDot=on  SenseZDDot=on  SenseRadDDot=off  SenseAzimDDot=off  SenseDistDDot=off  SenseIncDDot=off
  Transpose1 : Math  Commented=on  Operator=transpose  SignedPower=on  RndMeth=Zero  SaturateOnIntegerOverflow=on
  World Frame : sm_lib/Frames and Transforms/World Frame
  Wz : Outport  VectorParamsAs1DForOutWhenUnconnected=off
  Wx : Outport  Port=2  VectorParamsAs1DForOutWhenUnconnected=off
  Wy : Outport  Port=3  VectorParamsAs1DForOutWhenUnconnected=off
  ax : Outport  Port=4  VectorParamsAs1DForOutWhenUnconnected=off
  ay : Outport  Port=5  VectorParamsAs1DForOutWhenUnconnected=off
  az : Outport  Port=6  VectorParamsAs1DForOutWhenUnconnected=off
  wires:
  PS-Simulink Converter1/1 -> Wx/1
  PS-Simulink Converter/1 -> Wz/1
  PS-Simulink Converter2/1 -> Wy/1
  PS-Simulink Converter6/1 -> Transpose1/1
  PS-Simulink Converter7/1 -> Mux/1
  PS-Simulink Converter8/1 -> Mux/2
  PS-Simulink Converter9/1 -> Mux/3  "ax Imu"
  Mux/1 -> Product/2, Display2/1
  PS-Simulink Converter10/1 -> Mux2/1
  PS-Simulink Converter11/1 -> Mux2/2
  PS-Simulink Converter12/1 -> Mux2/3
  From1/1 -> Product1/1
  Product1/1 -> Scope13/1, Display4/1
  Mux2/1 -> Product1/2
  Transpose1/1 -> Goto4/1
  From/1 -> Product/1
  Product/1 -> Display1/1, Demux/1
  Demux/1 -> Scope2/1
  Demux/2 -> Scope3/1
  From8/1 -> Scope3/2
  Demux/3 -> Scope4/1
  From5/1 -> Scope4/2
  From7/1 -> Scope2/2
  YAW/1 -> Subsystem4/1(theta)
  PItch/1 -> Subsystem1/1(theta)
  "roll "/1 -> Subsystem2/1(theta)
  PS-Simulink Converter4/1 -> MATLAB Function/2(pitch)
  PS-Simulink Converter3/1 -> MATLAB Function/1(yaw)
  PS-Simulink Converter5/1 -> MATLAB Function/3(roll)
  Gain/1 -> Subsystem3/1(theta)
  Sine Wave1/1 -> Gain/1
  Sine Wave2/1 -> Gain1/1
  Gain1/1 -> Subsystem5/1(theta)
  Gain2/1 -> Subsystem6/1(theta)
  Sine Wave3/1 -> Gain2/1
  PS-Simulink Converter13/1 -> [ax], Scope/1
  PS-Simulink Converter14/1 -> Scope6/1, [ay], Scope1/1  "ay"
  PS-Simulink Converter15/1 -> Scope6/2, [az], Scope5/1  "az"
  Sum/1 -> ax/1
  MATLAB Function/1(ax) -> Sum/1
  [ax] -> Sum/2
  MATLAB Function/3(az) -> Sum1/1
  Sum1/1 -> az/1
  [az] -> Sum1/2
  Sum2/1 -> ay/1
  [ay] -> Sum2/2
  MATLAB Function/2(ay) -> Sum2/1
  connections:
  Subsystem2/RConn1 -- Revolute Joint X/LConn2
  Transform Sensor/RConn7 -- PS-Simulink Converter11/LConn1
  PS-Simulink Converter6/LConn1 -- Transform Sensor/RConn2
  PS-Simulink Converter8/LConn1 -- Transform Sensor/RConn4
  PS-Simulink Converter9/LConn1 -- Transform Sensor/RConn5
  PS-Simulink Converter10/LConn1 -- Transform Sensor/RConn6
  PS-Simulink Converter7/LConn1 -- Transform Sensor/RConn3
  Rigid Transform/LConn1 -- Revolute Joint Z/RConn1
  Revolute Joint Y/LConn1 -- Rigid Transform/RConn1
  Revolute Joint Y/RConn1 -- Rigid Transform1/LConn1
  Transform Sensor/RConn1 -- Rigid Transform3/RConn1 -- Solid/RConn1
  Rigid Transform1/RConn1 -- Revolute Joint X/LConn1
  Revolute Joint X/RConn1 -- Rigid Transform2/LConn1
  Rigid Transform2/RConn1 -- Rigid Transform3/LConn1
  PS-Simulink Converter12/LConn1 -- Transform Sensor/RConn8
  Subsystem4/RConn1 -- Revolute Joint Z/LConn2
  Subsystem1/RConn1 -- Revolute Joint Y/LConn2
  Revolute Joint Z/RConn3 -- PS-Simulink Converter/LConn1
  Revolute Joint Z/RConn2 -- PS-Simulink Converter3/LConn1
  Revolute Joint Y/RConn3 -- PS-Simulink Converter2/LConn1
  Revolute Joint Y/RConn2 -- PS-Simulink Converter4/LConn1
  Revolute Joint X/RConn3 -- PS-Simulink Converter1/LConn1
  Revolute Joint X/RConn2 -- PS-Simulink Converter5/LConn1
  Cartesian Joint/RConn1 -- Revolute Joint Z/LConn1
  Subsystem3/RConn1 -- Cartesian Joint/LConn2
  Subsystem5/RConn1 -- Cartesian Joint/LConn3
  Subsystem6/RConn1 -- Cartesian Joint/LConn4
  Solver Configuration/RConn1 -- Rigid Transform4/LConn1 -- Cartesian Joint/LConn1 -- World Frame/RConn1 -- Mechanism Configuration/RConn1
  Solid1/RConn1 -- Rigid Transform4/RConn1
  PS-Simulink Converter13/LConn1 -- Cartesian Joint/RConn2
  PS-Simulink Converter14/LConn1 -- Cartesian Joint/RConn3
  PS-Simulink Converter15/LConn1 -- Cartesian Joint/RConn4

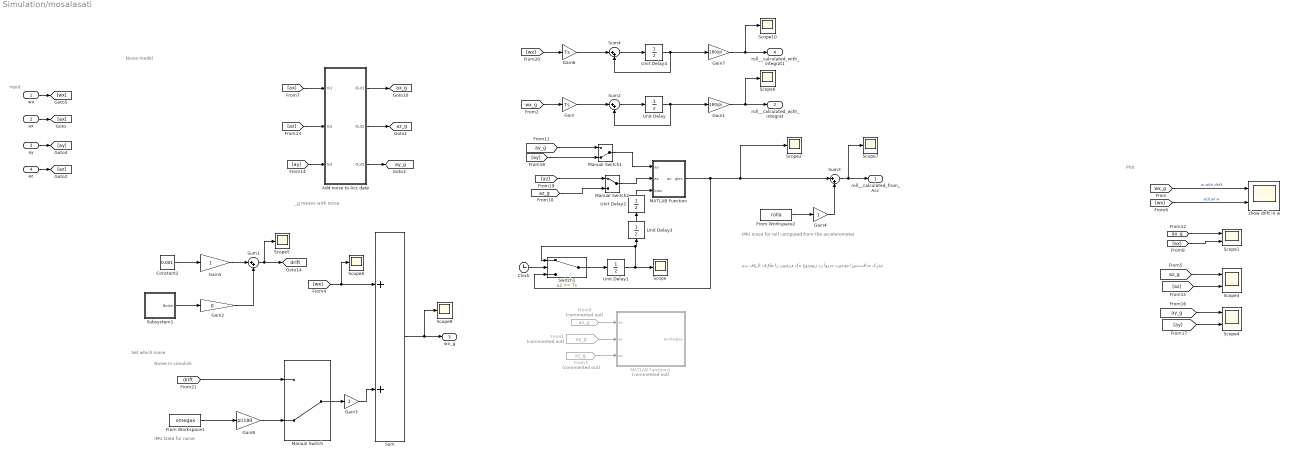
== system Simulation/mosalasati ==
  note: Set which niose
  note: Input
  note: Plot
  note: Noise model
  note: _g means with noise
  note: IMU Date for noise
  note: Niose in simulink
  note: IMU niose for roll computed
      | from the accelerometer
  note: من فعلا فقط از نویزی که خودمون در آورده بودیم
      | استفاده کردم
  wx : Inport
  ax : Inport  Port=2
  ay : Inport  Port=3
  az : Inport  Port=4
  Add noise to Acc date : Subsystem
  Clock : Clock
  Constant2 : Constant  Value=0.001
  From Workspace1 : FromWorkspace  VariableName=omegax  SampleTime=-1
  From Workspace2 : FromWorkspace  VariableName=rolla  SampleTime=-1
  From1 : From  Commented=on  GotoTag=ay_g  TagVisibility=global
  From3 : From  Commented=on  GotoTag=az_g  TagVisibility=global
  From9 : From  Commented=on  GotoTag=ax_g  TagVisibility=global
  Gain : Gain  Gain=Ts
  Gain1 : Gain  Gain=180/pi
  Gain2 : Gain  Gain=0
  Gain3 : Gain
  Gain4 : Gain
  Gain5 : Gain
  Gain6 : Gain  Gain=Ts
  Gain7 : Gain  Gain=180/pi
  Gain8 : Gain  Gain=pi/180
  MATLAB Function : MATLAB Function  TreatAsAtomicUnit=on
  MATLAB Function1 : MATLAB Function  Commented=on  TreatAsAtomicUnit=on
  Manual Switch : ManualSwitch  CurrentSetting=0
  Manual Switch1 : ManualSwitch  CurrentSetting=0
  Manual Switch2 : ManualSwitch
  Scope{,2,5..10} (8 alike) : Scope
  Scope1 : Scope  NumInputPorts=2
  Scope3 : Scope  NumInputPorts=2
  Scope4 : Scope  NumInputPorts=2
  Subsystem1 : Subsystem
  Sum : Sum
  Sum{1..4} (4 alike) : Sum  Inputs=|++
  Switch1 : Switch  Threshold=Ts
  Unit Delay{,1..4} (5 alike) : UnitDelay  SampleTime=-1  HasFrameUpgradeWarning=on
  show drift in w : Scope  NumInputPorts=2
  roll__calculated_from_Acc : Outport  VectorParamsAs1DForOutWhenUnconnected=off
  roll__calculated_with_integrat : Outport  Port=2  VectorParamsAs1DForOutWhenUnconnected=off
  wx_g : Outport  Port=3  VectorParamsAs1DForOutWhenUnconnected=off
  roll__calculated_with_integrat1 : Outport  Port=4  VectorParamsAs1DForOutWhenUnconnected=off
  tag scope: ax_g=global, ay_g=global, az_g=global, drift=global
  wires:
  [wx_g] -> Gain/1
  Unit Delay/1 -> Gain1/1, Sum2/2
  Gain/1 -> Sum2/1
  Sum2/1 -> Unit Delay/1
  From9/1 -> MATLAB Function1/1(ax)
  From1/1 -> MATLAB Function1/2(ay)
  From3/1 -> MATLAB Function1/3(az)
  MATLAB Function/1(accAnglex) -> Switch1/3, Sum3/1, Scope2/1
  Clock/1 -> Switch1/2
  Switch1/1 -> Unit Delay1/1
  Unit Delay1/1 -> Scope/1, Switch1/1, Unit Delay3/1
  Unit Delay2/1 -> MATLAB Function/3(bias)
  Unit Delay3/1 -> Unit Delay2/1
  Add noise to Acc date/1(Out1) -> [ax_g]
  [ay] -> Add noise to Acc date/3(In3)
  [az] -> Add noise to Acc date/2(In2)
  [ax] -> Add noise to Acc date/1(In1)
  Add noise to Acc date/3(Out3) -> [ay_g]
  Add noise to Acc date/2(Out2) -> [az_g]
  Subsystem1/1(Noise) -> Gain2/1
  [wx] -> Scope8/1, Sum/1
  Gain2/1 -> Sum1/2
  Gain5/1 -> Sum1/1
  Gain3/1 -> Sum/2
  Sum1/1 -> Scope5/1, [drift]
  Constant2/1 -> Gain5/1
  Gain1/1 -> Scope6/1, roll__calculated_with_integrat/1
  [wx_g] -> show drift in w/1  "w with drift"
  [wx] -> show drift in w/2  "actual w"
  [az_g] -> Scope3/1
  [ax] -> Scope1/2
  [ax_g] -> Scope1/1
  [az] -> Scope3/2
  [ay_g] -> Scope4/1
  [ay] -> Scope4/2
  Sum/1 -> Scope9/1, wx_g/1
  wx/1 -> [wx]
  ay/1 -> [ay]
  az/1 -> [az]
  ax/1 -> [ax]
  [drift] -> Manual Switch/1
  Manual Switch/1 -> Gain3/1
  From Workspace1/1 -> Gain8/1
  Sum3/1 -> Scope7/1, roll__calculated_from_Acc/1
  From Workspace2/1 -> Gain4/1
  Gain4/1 -> Sum3/2
  Manual Switch1/1 -> MATLAB Function/1(ay)
  [ay] -> Manual Switch1/2
  [ay_g] -> Manual Switch1/1
  Manual Switch2/1 -> MATLAB Function/2(az)
  [az] -> Manual Switch2/1
  [az_g] -> Manual Switch2/2
  Gain7/1 -> roll__calculated_with_integrat1/1, Scope10/1
  Sum4/1 -> Unit Delay4/1
  Gain6/1 -> Sum4/1
  Unit Delay4/1 -> Sum4/2, Gain7/1
  [wx] -> Gain6/1
  Gain8/1 -> Manual Switch/2

== system Simulation/Simscape Model/Subsystem1 ==
  theta : Inport
  Derivative : Derivative
  Derivative1 : Derivative
  Simulink-PS Converter : nesl_utility/Simulink-PS Converter  PhysicalDomain=network_engine_domain  SubClassName=ps_input  LeftPortType=input  RightPortType=output  PseudoPeriodic=off  Frequencies=[]  NoiseDistribution=none  NoiseParameters=[]  Unit=1  AffineConversion=off  FilteringAndDerivatives=provide  SimscapeFilterOrder=1  InputFilterTimeConstant=0.001  UdotUserProvided=2
      settings: SourceProductBaseCode=PW,SS
  Conn1 : PMIOPort  Side=Right
  wires:
  Derivative1/1 -> Simulink-PS Converter/3
  Derivative/1 -> Derivative1/1, Simulink-PS Converter/2
  theta/1 -> Derivative/1, Simulink-PS Converter/1
  connections:
  Simulink-PS Converter/RConn1 -- Conn1/RConn1

== system Simulation/Simscape Model/Subsystem2 ==
  theta : Inport
  Derivative : Derivative
  Derivative1 : Derivative
  Simulink-PS Converter : nesl_utility/Simulink-PS Converter  PhysicalDomain=network_engine_domain  SubClassName=ps_input  LeftPortType=input  RightPortType=output  PseudoPeriodic=off  Frequencies=[]  NoiseDistribution=none  NoiseParameters=[]  Unit=1  AffineConversion=off  FilteringAndDerivatives=provide  SimscapeFilterOrder=1  InputFilterTimeConstant=0.001  UdotUserProvided=2
      settings: SourceProductBaseCode=PW,SS
  Conn1 : PMIOPort  Side=Right
  wires:
  theta/1 -> Simulink-PS Converter/1, Derivative/1
  Derivative/1 -> Simulink-PS Converter/2, Derivative1/1
  Derivative1/1 -> Simulink-PS Converter/3
  connections:
  Simulink-PS Converter/RConn1 -- Conn1/RConn1

== system Simulation/Simscape Model/Subsystem3 ==
  theta : Inport
  Derivative : Derivative
  Derivative1 : Derivative
  Simulink-PS Converter : nesl_utility/Simulink-PS Converter  PhysicalDomain=network_engine_domain  SubClassName=ps_input  LeftPortType=input  RightPortType=output  PseudoPeriodic=off  Frequencies=[]  NoiseDistribution=none  NoiseParameters=[]  Unit=1  AffineConversion=off  FilteringAndDerivatives=provide  SimscapeFilterOrder=1  InputFilterTimeConstant=0.001  UdotUserProvided=2
      settings: SourceProductBaseCode=PW,SS
  Conn1 : PMIOPort  Side=Right
  wires:
  Derivative1/1 -> Simulink-PS Converter/3
  Derivative/1 -> Derivative1/1, Simulink-PS Converter/2
  theta/1 -> Derivative/1, Simulink-PS Converter/1
  connections:
  Simulink-PS Converter/RConn1 -- Conn1/RConn1

== system Simulation/Simscape Model/Subsystem4 ==
  theta : Inport
  Derivative : Derivative
  Derivative1 : Derivative
  Simulink-PS Converter : nesl_utility/Simulink-PS Converter  PhysicalDomain=network_engine_domain  SubClassName=ps_input  LeftPortType=input  RightPortType=output  PseudoPeriodic=off  Frequencies=[]  NoiseDistribution=none  NoiseParameters=[]  Unit=1  AffineConversion=off  FilteringAndDerivatives=provide  SimscapeFilterOrder=1  InputFilterTimeConstant=0.001  UdotUserProvided=2
      settings: SourceProductBaseCode=PW,SS
  Conn1 : PMIOPort  Side=Right
  wires:
  theta/1 -> Simulink-PS Converter/1, Derivative/1
  Derivative/1 -> Simulink-PS Converter/2, Derivative1/1
  Derivative1/1 -> Simulink-PS Converter/3
  connections:
  Simulink-PS Converter/RConn1 -- Conn1/RConn1

== system Simulation/Simscape Model/Subsystem5 ==
  theta : Inport
  Derivative : Derivative
  Derivative1 : Derivative
  Simulink-PS Converter : nesl_utility/Simulink-PS Converter  PhysicalDomain=network_engine_domain  SubClassName=ps_input  LeftPortType=input  RightPortType=output  PseudoPeriodic=off  Frequencies=[]  NoiseDistribution=none  NoiseParameters=[]  Unit=1  AffineConversion=off  FilteringAndDerivatives=provide  SimscapeFilterOrder=1  InputFilterTimeConstant=0.001  UdotUserProvided=2
      settings: SourceProductBaseCode=PW,SS
  Conn1 : PMIOPort  Side=Right
  wires:
  theta/1 -> Simulink-PS Converter/1, Derivative/1
  Derivative/1 -> Simulink-PS Converter/2, Derivative1/1
  Derivative1/1 -> Simulink-PS Converter/3
  connections:
  Simulink-PS Converter/RConn1 -- Conn1/RConn1

== system Simulation/Simscape Model/Subsystem6 ==
  theta : Inport
  Derivative : Derivative
  Derivative1 : Derivative
  Simulink-PS Converter : nesl_utility/Simulink-PS Converter  PhysicalDomain=network_engine_domain  SubClassName=ps_input  LeftPortType=input  RightPortType=output  PseudoPeriodic=off  Frequencies=[]  NoiseDistribution=none  NoiseParameters=[]  Unit=1  AffineConversion=off  FilteringAndDerivatives=provide  SimscapeFilterOrder=1  InputFilterTimeConstant=0.001  UdotUserProvided=2
      settings: SourceProductBaseCode=PW,SS
  Conn1 : PMIOPort  Side=Right
  wires:
  Derivative1/1 -> Simulink-PS Converter/3
  Derivative/1 -> Derivative1/1, Simulink-PS Converter/2
  theta/1 -> Derivative/1, Simulink-PS Converter/1
  connections:
  Simulink-PS Converter/RConn1 -- Conn1/RConn1
